simulink model "BOOST_COMPLETE_MODEL_WITH"  (R2024b)
settings: Solver=VariableStepAuto  StartTime=0.0  StopTime=10.0  RelTol=1e-3
values from neighbouring files (symbols this model uses):
  beta = Rb/(Ra+Rb)    (= 0.25)    [AUTO_TUNE.m]
  D_dash = Vi/Vo    (= 0.4)    [AUTO_TUNE.m]
  r = 0.002    [AUTO_TUNE.m]
  Ra = 30e3    (= 30000)    [AUTO_TUNE.m]
  Rb = 10e3    (= 10000)    [AUTO_TUNE.m]
  Rc = 0.001    [AUTO_TUNE.m]
  Tm = 1    [AUTO_TUNE.m]    (also in code_pi.m)
  Vi = 48    [AUTO_TUNE.m]
undefined symbols (not defined in the file or in its folder): den, num
libraries: spsParallelRLCBranchLib x7, spsVoltageMeasurementLib x4, spsCurrentMeasurementLib x3, spsSawtoothGeneratorLib x2, spsDCVoltageSourceLib x1, spsDiodeLib x1, spsMosfetLib x1, spspowerguiLib x1
settings Model: Creator=S SURYA  LastModifiedBy=S SURYA

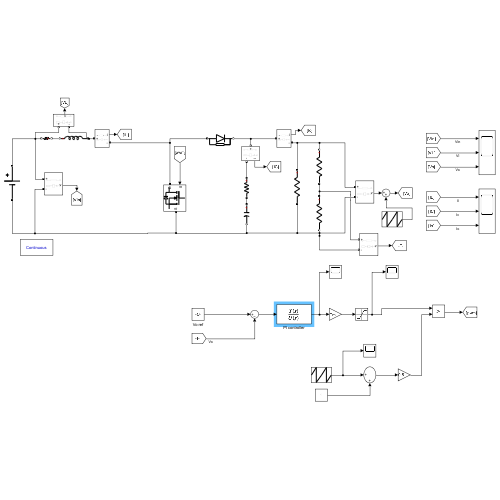
[thumbnail: Simulink's stored preview of the top-level diagram]
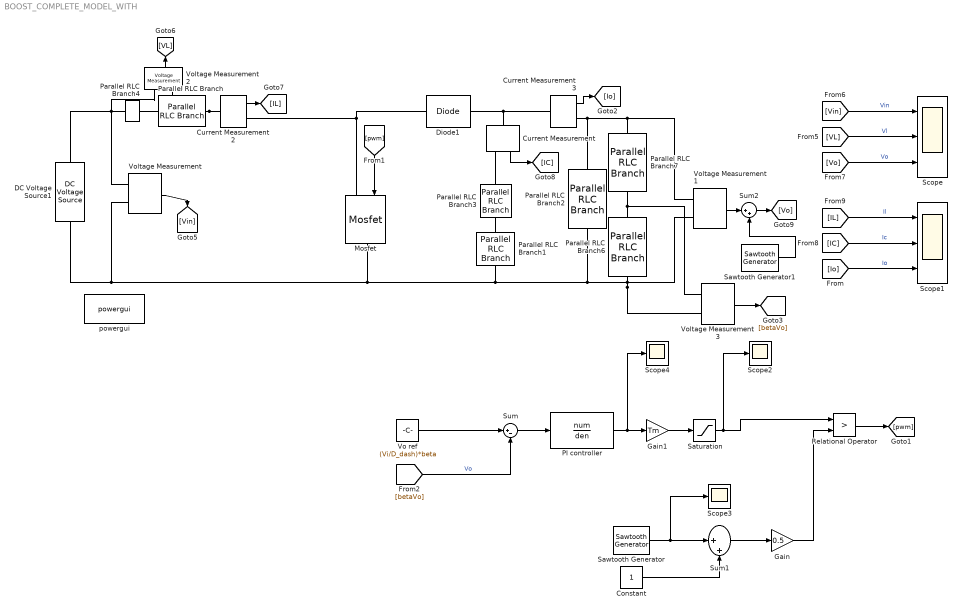
== system BOOST_COMPLETE_MODEL_WITH ==
  Constant : Constant
  Current Measurement : spsCurrentMeasurementLib/Current Measurement  PhasorSimulation=off  OutputType=Complex  PSBequivalent=0
  Current Measurement2 : spsCurrentMeasurementLib/Current Measurement  PhasorSimulation=off  OutputType=Complex  PSBequivalent=0
  Current Measurement3 : spsCurrentMeasurementLib/Current Measurement  PhasorSimulation=off  OutputType=Complex  PSBequivalent=0
  DC Voltage Source1 : spsDCVoltageSourceLib/DC Voltage Source  Amplitude=48  Measurements=None
  Diode1 : spsDiodeLib/Diode  Ron=0.0001  Lon=0  Vf=0.8  IC=0  UseSnubber=0  Rs=500  Cs=250e-9  Measurements=off
  Gain : Gain  Gain=0.5
  Gain1 : Gain  Gain=Tm
  Mosfet : spsMosfetLib/Mosfet  Ron=0.1  Lon=0  Rd=0.01  Vfd=0  IC=0  Rs=1e5  Cs=inf  Measurements=off
  PI controller : TransferFcn  Numerator=num  Denominator=den
  Parallel RLC Branch : spsParallelRLCBranchLib/Parallel RLC Branch  LConnTagsString=a  RConnTagsString=__new0  BranchType=L  Resistance=1  Inductance=200e-6  SetiL0=off  InitialCurrent=0  Capacitance=1e-6  Setx0=off  InitialVoltage=0  Measurements=None
  Parallel RLC Branch1 : spsParallelRLCBranchLib/Parallel RLC Branch  LConnTagsString=a  RConnTagsString=__new0  BranchType=C  Resistance=1  Inductance=200e-6  SetiL0=off  InitialCurrent=0  Capacitance=33e-6  Setx0=off  InitialVoltage=0  Measurements=None
  Parallel RLC Branch2 : spsParallelRLCBranchLib/Parallel RLC Branch  LConnTagsString=a  RConnTagsString=__new0  BranchType=R  Resistance=12  Inductance=200e-6  SetiL0=off  InitialCurrent=0  Capacitance=1e-6  Setx0=off  InitialVoltage=0  Measurements=None
  Parallel RLC Branch3 : spsParallelRLCBranchLib/Parallel RLC Branch  LConnTagsString=a  RConnTagsString=__new0  BranchType=R  Resistance=Rc  Inductance=200e-6  SetiL0=off  InitialCurrent=0  Capacitance=1e-6  Setx0=off  InitialVoltage=0  Measurements=None
  Parallel RLC Branch4 : spsParallelRLCBranchLib/Parallel RLC Branch  LConnTagsString=a  RConnTagsString=__new0  BranchType=R  Resistance=r  Inductance=200e-6  SetiL0=off  InitialCurrent=0  Capacitance=1e-6  Setx0=off  InitialVoltage=0  Measurements=None
  Parallel RLC Branch6 : spsParallelRLCBranchLib/Parallel RLC Branch  LConnTagsString=a  RConnTagsString=__new0  BranchType=R  Resistance=Rb  Inductance=200e-6  SetiL0=off  InitialCurrent=0  Capacitance=1e-6  Setx0=off  InitialVoltage=0  Measurements=None
  Parallel RLC Branch7 : spsParallelRLCBranchLib/Parallel RLC Branch  LConnTagsString=a  RConnTagsString=__new0  BranchType=R  Resistance=Ra  Inductance=200e-6  SetiL0=off  InitialCurrent=0  Capacitance=1e-6  Setx0=off  InitialVoltage=0  Measurements=None
  Relational Operator : RelationalOperator  Operator=>  OutDataTypeStr=boolean  RndMeth=Simplest  InputSameDT=off
  Saturation : Saturate  UpperLimit=1  LowerLimit=-1
  Sawtooth Generator : spsSawtoothGeneratorLib/Sawtooth Generator  Freq=200e3  Phase=180  Ts=0
  Sawtooth Generator1 : spsSawtoothGeneratorLib/Sawtooth Generator  Freq=200e3  Phase=180  Ts=0
  Scope : Scope  NumInputPorts=3
  Scope1 : Scope  NumInputPorts=3
  Scope2 : Scope
  Scope3 : Scope
  Scope4 : Scope
  Sum : Sum  Inputs=|+-
  Sum1 : Sum  Inputs=|++
  Sum2 : Sum  Inputs=|++
  Vo ref : Constant  Value=(Vi/D_dash)*beta
  Voltage Measurement{,1..3} (4 alike) : spsVoltageMeasurementLib/Voltage Measurement  PhasorSimulation=off  OutputType=Complex  PSBequivalent=0
  powergui : spspowerguiLib/powergui  Priority=1  SimulationMode=Continuous  SampleTime=5e-6  frequency=60  Iterations=50  frequencyindice=0  Pbase=100e6  ErrMax=1e-4  UnitsV=kV  UnitsW=MW  buscounter=0  FunctionMessages=off  echomessages=off  EnableUseOfTLC=off  CurrentSourceSwitches=off  DisableSnubberDevices=off  DisableRonSwitches=off  DisableVfSwitches=off  DisplayEquations=off  AutomaticDiscreteSolvers=off  SolverType=Tustin/Backward Euler (TBE)  Interpol=off  ExternalGateDelay=off  methode=off  Ts=100  x0status=blocks  SPID=on  SwTol=0  HookPort=off  NonlinearTolerance=1e-4  nMaxIteration=100  ContinueOnMaxIteration=off  RestoreLinks=warning  ResistiveCurrentMeasurement=off  Frange=[0:2:500]  Ylog=off  Xlog=on  ShowGrid=off  save=off  variable=ZData  structure=0  ZoomFFT=off  StartTime=0.0  cycles=1  DisplayStyle=1  fundamental=60  FreqAxis=off  MaxFrequency=1000  frequencyindicesteady=1  RmsSteady=1  display=off
  wires:
  [pwm] -> Mosfet/1
  Vo ref/1 -> Sum/1
  Relational Operator/1 -> [pwm]
  Constant/1 -> Sum1/2
  Current Measurement/1 -> [IC]
  [Io] -> Scope1/3  "Io"
  Voltage Measurement/1 -> [Vin]
  PI controller/1 -> Scope4/1, Gain1/1
  Gain/1 -> Relational Operator/2
  Voltage Measurement1/1 -> Sum2/1
  Gain1/1 -> Saturation/1
  Sum2/1 -> [Vo]
  Sum1/1 -> Gain/1
  Sawtooth Generator/1 -> Scope3/1, Sum1/1
  Current Measurement2/1 -> [IL]
  Sum/1 -> PI controller/1
  Voltage Measurement3/1 -> [betaVo]
  [IL] -> Scope1/1  "Il"
  Current Measurement3/1 -> [Io]
  [betaVo] -> Sum/2  "Vo"
  [VL] -> Scope/2  "Vl"
  [Vin] -> Scope/1  "Vin"
  [Vo] -> Scope/3  "Vo"
  Saturation/1 -> Scope2/1, Relational Operator/1
  Voltage Measurement2/1 -> [VL]
  Sawtooth Generator1/1 -> Sum2/2
  [IC] -> Scope1/2  "Ic"
  connections:
  Voltage Measurement2/LConn1 -- DC Voltage Source1/RConn1 -- Parallel RLC Branch4/RConn1 -- Voltage Measurement/LConn1
  Parallel RLC Branch2/LConn1 -- Voltage Measurement1/LConn1 -- Parallel RLC Branch7/LConn1 -- Current Measurement3/RConn1
  Current Measurement/LConn1 -- Diode1/RConn1 -- Current Measurement3/LConn1
  Parallel RLC Branch1/RConn1 -- Voltage Measurement/LConn2 -- DC Voltage Source1/LConn1 -- Mosfet/RConn1 -- Voltage Measurement3/LConn2 -- Parallel RLC Branch6/RConn1 -- Voltage Measurement1/LConn2 -- Parallel RLC Branch2/RConn1
  Parallel RLC Branch6/LConn1 -- Parallel RLC Branch7/RConn1 -- Voltage Measurement3/LConn1
  Current Measurement2/LConn1 -- Parallel RLC Branch/RConn1 -- Voltage Measurement2/LConn2
  Mosfet/LConn1 -- Diode1/LConn1 -- Current Measurement2/RConn1
  Parallel RLC Branch/LConn1 -- Parallel RLC Branch4/LConn1
  Parallel RLC Branch3/RConn1 -- Parallel RLC Branch1/LConn1
  Current Measurement/RConn1 -- Parallel RLC Branch3/LConn1
